simulink model "Simulink_EI"  (R2024b)
settings: Solver=ode23tb  StartTime=0.0  StopTime=20  FixedStep=0.00694  RelTol=1e-3
values from neighbouring files (symbols this model uses):
  beta = 1/1820.89    (= 0.000549181993421)    [Matlab_EI_1.m]
  Hco2 = 4003    [Matlab_EI_1.m]
  Ho2 = 94565    [Matlab_EI_1.m]
  phi = 0.2029    [Matlab_EI_1.m]
libraries: slpidlib x6
(part 1 of 2)
settings Model: Creator=julesmaugin  LastModifiedBy=julesmaugin

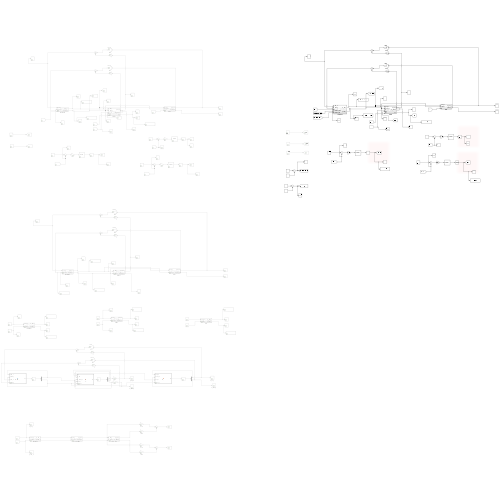
[thumbnail: Simulink's stored preview of the top-level diagram]
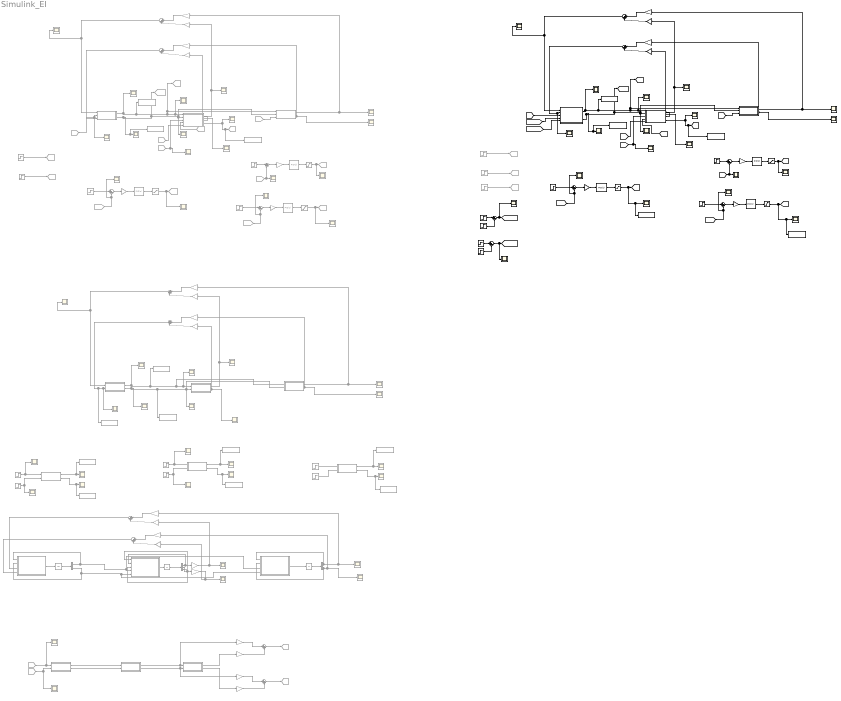
== system Simulink_EI ==
  1-phi{,1,4..7} (6 alike) : Gain  Commented=on  Gain=1-phi
  1-phi2 : Gain  Commented=on  Gain=0.7971
  1-phi3 : Gain  Commented=on  Gain=0.7971
  1-phi8 : Gain  Gain=1-phi
  1-phi9 : Gain  Gain=1-phi
  Algue : Subsystem  Commented=on
  Algue1 : Subsystem  Commented=on
  Algue2 : Subsystem  Commented=on
  Algue3 : Subsystem
  Blé : Subsystem  Commented=on
  Blé1 : Subsystem  Commented=on
  Blé2 : Subsystem  Commented=on
  Blé3 : Subsystem
  "C-IV a : algue" : Subsystem  Commented=on
  "C-IV b : blé" : Subsystem  Commented=on
  Demux : Demux  Commented=on  Outputs=2
  Demux1 : Demux  Commented=on  Outputs=3
  Demux2 : Demux  Commented=on  Outputs=2
  From : From  Commented=on  GotoTag=PO2e
  From1 : From  Commented=on  GotoTag=PCO2e
  From2 : From  Commented=on  GotoTag=Cx
  From3 : From  Commented=on  GotoTag=Lr
  From4 : From  Commented=on  GotoTag=P_CO2_c
  From5 : From  Commented=on  GotoTag=phi0
  From6 : From  Commented=on  GotoTag=Gc
  From7 : From  Commented=on  GotoTag=Gc
  From8 : From  Commented=on  GotoTag=Gc
  From9 : From  Commented=on  GotoTag=P_O2_c
  Gain : Gain  Commented=on  Gain=-10
  Gain1 : Gain  Commented=on  Gain=-5
  Gain2 : Gain  Commented=on
  Gain3 : Gain  Gain=-10
  Gain4 : Gain  Gain=-200
  Gain5 : Gain  Gain=10
  Goto : Goto  Commented=on  GotoTag=PO2e
  Goto1 : Goto  Commented=on  GotoTag=PCO2e
  Goto14 : Goto  Commented=on  GotoTag=phi0
  Goto17 : Goto  Commented=on  GotoTag=Gc
  Goto18 : Goto  Commented=on  GotoTag=Lr
  Goto2 : Goto  Commented=on  GotoTag=Lr
  Goto3 : Goto  Commented=on  GotoTag=Cx
  Goto4 : Goto  Commented=on  GotoTag=phi0
  Goto5 : Goto  Commented=on  GotoTag=P_CO2_c
  Goto6 : Goto  Commented=on  GotoTag=phi0
  Goto7 : Goto  Commented=on  GotoTag=Gc
  Goto8 : Goto  Commented=on  GotoTag=P_O2_c
  Goto9 : Goto  Commented=on  GotoTag=Gc
  Habitacle : Subsystem  Commented=on
  Habitacle1 : Subsystem  Commented=on
  Habitacle2 : Subsystem  Commented=on
  Habitacle3 : Subsystem  Commented=on
  Habitacle4 : Subsystem
  Integrator Limited : Integrator  Commented=on  InitialCondition=[20000;40]  LimitOutput=on  LowerSaturationLimit=0
  Integrator Limited1 : Integrator  Commented=on  InitialCondition=[0.212;18.79;1]  LimitOutput=on  LowerSaturationLimit=0
  Integrator Limited2 : Integrator  Commented=on  InitialCondition=[20000;20]  LimitOutput=on  LowerSaturationLimit=0
  MATLAB Function : MATLAB Function  Commented=on  TreatAsAtomicUnit=on
  MATLAB Function1 : MATLAB Function  Commented=on  TreatAsAtomicUnit=on
  MATLAB Function2 : MATLAB Function  Commented=on  TreatAsAtomicUnit=on
  Multiply : Gain  Commented=on  Gain=Ho2
  Multiply1 : Gain  Commented=on  Gain=Hco2
  PID Controller : slpidlib/PID Controller  Commented=on  Controller=PID  Form=Parallel  TimeDomain=Continuous-time  UseExternalTs=off  SampleTime=-1  IntegratorMethod=Forward Euler  FilterMethod=Forward Euler  ControllerParametersSource=internal  P=1  I=1  UseKiTs=off  D=0  UseExternalDerivativeSource=off  N=100  UseFilter=on  TunerSelectOption=Transfer Function Based (PID Tuner App)  InitialConditionSource=internal  InitialConditionForIntegrator=0  InitialConditionForFilter=0  DifferentiatorICPrevScaledInput=0  ExternalReset=none  TrackingMode=off  Kt=1  LimitOutput=off  SatLimitsSource=internal  UpperSaturationLimit=inf  LowerSaturationLimit=-inf  LinearizeAsGain=on  AntiWindupMode=none  Kb=1  LimitIntegrator=off  UpperIntegratorSaturationLimit=inf  LowerIntegratorSaturationLimit=-inf  POutMin=[]  POutMax=[]  IOutMin=[]  IOutMax=[]  DOutMin=[]  DOutMax=[]  NOutMin=[]  NOutMax=[]  SumOutMin=[]  SumOutMax=[]  SaturationOutMin=[]  SaturationOutMax=[]  PParamMin=[]  PParamMax=[]  IParamMin=[]  IParamMax=[]  DParamMin=[]  DParamMax=[]  NParamMin=[]  NParamMax=[]  KbParamMin=[]  KbParamMax=[]  KtParamMin=[]  KtParamMax=[]  KbOutMin=[]  KbOutMax=[]  KtOutMin=[]  KtOutMax=[]  IntegratorOutMin=[]  IntegratorOutMax=[]  FilterOutMin=[]  FilterOutMax=[]  SumI1OutMin=[]  SumI1OutMax=[]  SumI2OutMin=[]  SumI2OutMax=[]  SumI3OutMin=[]  SumI3OutMax=[]  SumI4OutMin=[]  SumI4OutMax=[]  SumDOutMin=[]  SumDOutMax=[]  DifferentiatorOutMin=[]  DifferentiatorOutMax=[]  FilterDiffOutCoefMin=[]  FilterDiffOutCoefMax=[]  ReciprocalOutMin=[]  ReciprocalOutMax=[]  SumDenOutMin=[]  SumDenOutMax=[]  SumNumOutMin=[]  SumNumOutMax=[]  DivideOutMin=[]  DivideOutMax=[]  UdiffTsProdOutMin=[]  UdiffTsProdOutMax=[]  NTsProdOutMin=[]  NTsProdOutMax=[]  UintegralTsProdOutMin=[]  UintegralTsProdOutMax=[]  UngainTsProdOutMin=[]  UngainTsProdOutMax=[]  ClampingZeroOutDataTypeStr=Inherit: Inherit via back propagation  ClampingZeroOutMin=[]  ClampingZeroOutMax=[]  FilterDenConstantOutDataTypeStr=Inherit: Inherit via back propagation  FilterDenConstantOutMin=[]  FilterDenConstantOutMax=[]  PCopyOutDataTypeStr=Inherit: Inherit via back propagation  PCopyOutMin=[]  PCopyOutMax=[]  NCopyOutDataTypeStr=Inherit: Inherit via back propagation  NCopyOutMin=[]  NCopyOutMax=[]  IntegratorContinuousStateAttributes=''  IntegratorStateMustResolveToSignalObject=off  IntegratorRTWStateStorageClass=Auto  FilterContinuousStateAttributes=''  FilterStateMustResolveToSignalObject=off  FilterRTWStateStorageClass=Auto  ParallelPVariant=InternalParameters  IdealPVariant=Disabled  IVariant=InternalParameters  DVariant=InternalParameters  IntegratorVariant=Continuous  SatVariant=Disabled  AWVariant=Passthrough  PCopyVariant=Disabled  TRVariant=Disabled  FdbkBlocksVariant=Forward  IdealPFdbkVariant=Disabled  SatFdbkVariant=Disabled  DerivativeFilterVariant=ContFilter  NVariant=InternalParameters  NCopyVariant=Disabled  FilterICVariant=InternalICsFilter  IntegratorICVariant=InternalICs  ExternalResetVariant=Disabled  TRSumVariant=Passthrough  SumFdbkVariant=Disabled  SumVariant=Sum_PID  TsampFilterVariant=InternalTs  TsampNgainVariant=Passthrough  TsampIntegralVariant=Disabled_SignalSpec  ExternalSaturationOutDataTypeStr=Inherit: Same as second input  DerivativeSourceVariant=ErrorSignal  PreIntVariant=InternalPreInt
  PID Controller1 : slpidlib/PID Controller  Commented=on  Controller=PID  Form=Parallel  TimeDomain=Continuous-time  UseExternalTs=off  SampleTime=-1  IntegratorMethod=Forward Euler  FilterMethod=Forward Euler  ControllerParametersSource=internal  P=1  I=10  UseKiTs=off  D=0  UseExternalDerivativeSource=off  N=100  UseFilter=on  TunerSelectOption=Transfer Function Based (PID Tuner App)  InitialConditionSource=internal  InitialConditionForIntegrator=0  InitialConditionForFilter=0  DifferentiatorICPrevScaledInput=0  ExternalReset=none  TrackingMode=off  Kt=1  LimitOutput=off  SatLimitsSource=internal  UpperSaturationLimit=inf  LowerSaturationLimit=-inf  LinearizeAsGain=on  AntiWindupMode=none  Kb=1  LimitIntegrator=off  UpperIntegratorSaturationLimit=inf  LowerIntegratorSaturationLimit=-inf  POutMin=[]  POutMax=[]  IOutMin=[]  IOutMax=[]  DOutMin=[]  DOutMax=[]  NOutMin=[]  NOutMax=[]  SumOutMin=[]  SumOutMax=[]  SaturationOutMin=[]  SaturationOutMax=[]  PParamMin=[]  PParamMax=[]  IParamMin=[]  IParamMax=[]  DParamMin=[]  DParamMax=[]  NParamMin=[]  NParamMax=[]  KbParamMin=[]  KbParamMax=[]  KtParamMin=[]  KtParamMax=[]  KbOutMin=[]  KbOutMax=[]  KtOutMin=[]  KtOutMax=[]  IntegratorOutMin=[]  IntegratorOutMax=[]  FilterOutMin=[]  FilterOutMax=[]  SumI1OutMin=[]  SumI1OutMax=[]  SumI2OutMin=[]  SumI2OutMax=[]  SumI3OutMin=[]  SumI3OutMax=[]  SumI4OutMin=[]  SumI4OutMax=[]  SumDOutMin=[]  SumDOutMax=[]  DifferentiatorOutMin=[]  DifferentiatorOutMax=[]  FilterDiffOutCoefMin=[]  FilterDiffOutCoefMax=[]  ReciprocalOutMin=[]  ReciprocalOutMax=[]  SumDenOutMin=[]  SumDenOutMax=[]  SumNumOutMin=[]  SumNumOutMax=[]  DivideOutMin=[]  DivideOutMax=[]  UdiffTsProdOutMin=[]  UdiffTsProdOutMax=[]  NTsProdOutMin=[]  NTsProdOutMax=[]  UintegralTsProdOutMin=[]  UintegralTsProdOutMax=[]  UngainTsProdOutMin=[]  UngainTsProdOutMax=[]  ClampingZeroOutDataTypeStr=Inherit: Inherit via back propagation  ClampingZeroOutMin=[]  ClampingZeroOutMax=[]  FilterDenConstantOutDataTypeStr=Inherit: Inherit via back propagation  FilterDenConstantOutMin=[]  FilterDenConstantOutMax=[]  PCopyOutDataTypeStr=Inherit: Inherit via back propagation  PCopyOutMin=[]  PCopyOutMax=[]  NCopyOutDataTypeStr=Inherit: Inherit via back propagation  NCopyOutMin=[]  NCopyOutMax=[]  IntegratorContinuousStateAttributes=''  IntegratorStateMustResolveToSignalObject=off  IntegratorRTWStateStorageClass=Auto  FilterContinuousStateAttributes=''  FilterStateMustResolveToSignalObject=off  FilterRTWStateStorageClass=Auto  ParallelPVariant=InternalParameters  IdealPVariant=Disabled  IVariant=InternalParameters  DVariant=InternalParameters  IntegratorVariant=Continuous  SatVariant=Disabled  AWVariant=Passthrough  PCopyVariant=Disabled  TRVariant=Disabled  FdbkBlocksVariant=Forward  IdealPFdbkVariant=Disabled  SatFdbkVariant=Disabled  DerivativeFilterVariant=ContFilter  NVariant=InternalParameters  NCopyVariant=Disabled  FilterICVariant=InternalICsFilter  IntegratorICVariant=InternalICs  ExternalResetVariant=Disabled  TRSumVariant=Passthrough  SumFdbkVariant=Disabled  SumVariant=Sum_PID  TsampFilterVariant=InternalTs  TsampNgainVariant=Passthrough  TsampIntegralVariant=Disabled_SignalSpec  ExternalSaturationOutDataTypeStr=Inherit: Same as second input  DerivativeSourceVariant=ErrorSignal  PreIntVariant=InternalPreInt
  PID Controller2 : slpidlib/PID Controller  Commented=on  Controller=PID  Form=Parallel  TimeDomain=Continuous-time  UseExternalTs=off  SampleTime=-1  IntegratorMethod=Forward Euler  FilterMethod=Forward Euler  ControllerParametersSource=internal  P=1  I=0  UseKiTs=off  D=0  UseExternalDerivativeSource=off  N=100  UseFilter=on  TunerSelectOption=Transfer Function Based (PID Tuner App)  InitialConditionSource=internal  InitialConditionForIntegrator=0  InitialConditionForFilter=0  DifferentiatorICPrevScaledInput=0  ExternalReset=none  TrackingMode=off  Kt=1  LimitOutput=off  SatLimitsSource=internal  UpperSaturationLimit=inf  LowerSaturationLimit=-inf  LinearizeAsGain=on  AntiWindupMode=none  Kb=1  LimitIntegrator=off  UpperIntegratorSaturationLimit=inf  LowerIntegratorSaturationLimit=-inf  POutMin=[]  POutMax=[]  IOutMin=[]  IOutMax=[]  DOutMin=[]  DOutMax=[]  NOutMin=[]  NOutMax=[]  SumOutMin=[]  SumOutMax=[]  SaturationOutMin=[]  SaturationOutMax=[]  PParamMin=[]  PParamMax=[]  IParamMin=[]  IParamMax=[]  DParamMin=[]  DParamMax=[]  NParamMin=[]  NParamMax=[]  KbParamMin=[]  KbParamMax=[]  KtParamMin=[]  KtParamMax=[]  KbOutMin=[]  KbOutMax=[]  KtOutMin=[]  KtOutMax=[]  IntegratorOutMin=[]  IntegratorOutMax=[]  FilterOutMin=[]  FilterOutMax=[]  SumI1OutMin=[]  SumI1OutMax=[]  SumI2OutMin=[]  SumI2OutMax=[]  SumI3OutMin=[]  SumI3OutMax=[]  SumI4OutMin=[]  SumI4OutMax=[]  SumDOutMin=[]  SumDOutMax=[]  DifferentiatorOutMin=[]  DifferentiatorOutMax=[]  FilterDiffOutCoefMin=[]  FilterDiffOutCoefMax=[]  ReciprocalOutMin=[]  ReciprocalOutMax=[]  SumDenOutMin=[]  SumDenOutMax=[]  SumNumOutMin=[]  SumNumOutMax=[]  DivideOutMin=[]  DivideOutMax=[]  UdiffTsProdOutMin=[]  UdiffTsProdOutMax=[]  NTsProdOutMin=[]  NTsProdOutMax=[]  UintegralTsProdOutMin=[]  UintegralTsProdOutMax=[]  UngainTsProdOutMin=[]  UngainTsProdOutMax=[]  ClampingZeroOutDataTypeStr=Inherit: Inherit via back propagation  ClampingZeroOutMin=[]  ClampingZeroOutMax=[]  FilterDenConstantOutDataTypeStr=Inherit: Inherit via back propagation  FilterDenConstantOutMin=[]  FilterDenConstantOutMax=[]  PCopyOutDataTypeStr=Inherit: Inherit via back propagation  PCopyOutMin=[]  PCopyOutMax=[]  NCopyOutDataTypeStr=Inherit: Inherit via back propagation  NCopyOutMin=[]  NCopyOutMax=[]  IntegratorContinuousStateAttributes=''  IntegratorStateMustResolveToSignalObject=off  IntegratorRTWStateStorageClass=Auto  FilterContinuousStateAttributes=''  FilterStateMustResolveToSignalObject=off  FilterRTWStateStorageClass=Auto  ParallelPVariant=InternalParameters  IdealPVariant=Disabled  IVariant=InternalParameters  DVariant=InternalParameters  IntegratorVariant=Continuous  SatVariant=Disabled  AWVariant=Passthrough  PCopyVariant=Disabled  TRVariant=Disabled  FdbkBlocksVariant=Forward  IdealPFdbkVariant=Disabled  SatFdbkVariant=Disabled  DerivativeFilterVariant=ContFilter  NVariant=InternalParameters  NCopyVariant=Disabled  FilterICVariant=InternalICsFilter  IntegratorICVariant=InternalICs  ExternalResetVariant=Disabled  TRSumVariant=Passthrough  SumFdbkVariant=Disabled  SumVariant=Sum_PID  TsampFilterVariant=InternalTs  TsampNgainVariant=Passthrough  TsampIntegralVariant=Disabled_SignalSpec  ExternalSaturationOutDataTypeStr=Inherit: Same as second input  DerivativeSourceVariant=ErrorSignal  PreIntVariant=InternalPreInt
  PID Controller3 : slpidlib/PID Controller  Controller=PID  Form=Parallel  TimeDomain=Continuous-time  UseExternalTs=off  SampleTime=-1  IntegratorMethod=Forward Euler  FilterMethod=Forward Euler  ControllerParametersSource=internal  P=1  I=1  UseKiTs=off  D=0  UseExternalDerivativeSource=off  N=100  UseFilter=on  TunerSelectOption=Transfer Function Based (PID Tuner App)  InitialConditionSource=internal  InitialConditionForIntegrator=0  InitialConditionForFilter=0  DifferentiatorICPrevScaledInput=0  ExternalReset=none  TrackingMode=off  Kt=1  LimitOutput=off  SatLimitsSource=internal  UpperSaturationLimit=inf  LowerSaturationLimit=-inf  LinearizeAsGain=on  AntiWindupMode=none  Kb=1  LimitIntegrator=off  UpperIntegratorSaturationLimit=inf  LowerIntegratorSaturationLimit=-inf  POutMin=[]  POutMax=[]  IOutMin=[]  IOutMax=[]  DOutMin=[]  DOutMax=[]  NOutMin=[]  NOutMax=[]  SumOutMin=[]  SumOutMax=[]  SaturationOutMin=[]  SaturationOutMax=[]  PParamMin=[]  PParamMax=[]  IParamMin=[]  IParamMax=[]  DParamMin=[]  DParamMax=[]  NParamMin=[]  NParamMax=[]  KbParamMin=[]  KbParamMax=[]  KtParamMin=[]  KtParamMax=[]  KbOutMin=[]  KbOutMax=[]  KtOutMin=[]  KtOutMax=[]  IntegratorOutMin=[]  IntegratorOutMax=[]  FilterOutMin=[]  FilterOutMax=[]  SumI1OutMin=[]  SumI1OutMax=[]  SumI2OutMin=[]  SumI2OutMax=[]  SumI3OutMin=[]  SumI3OutMax=[]  SumI4OutMin=[]  SumI4OutMax=[]  SumDOutMin=[]  SumDOutMax=[]  DifferentiatorOutMin=[]  DifferentiatorOutMax=[]  FilterDiffOutCoefMin=[]  FilterDiffOutCoefMax=[]  ReciprocalOutMin=[]  ReciprocalOutMax=[]  SumDenOutMin=[]  SumDenOutMax=[]  SumNumOutMin=[]  SumNumOutMax=[]  DivideOutMin=[]  DivideOutMax=[]  UdiffTsProdOutMin=[]  UdiffTsProdOutMax=[]  NTsProdOutMin=[]  NTsProdOutMax=[]  UintegralTsProdOutMin=[]  UintegralTsProdOutMax=[]  UngainTsProdOutMin=[]  UngainTsProdOutMax=[]  ClampingZeroOutDataTypeStr=Inherit: Inherit via back propagation  ClampingZeroOutMin=[]  ClampingZeroOutMax=[]  FilterDenConstantOutDataTypeStr=Inherit: Inherit via back propagation  FilterDenConstantOutMin=[]  FilterDenConstantOutMax=[]  PCopyOutDataTypeStr=Inherit: Inherit via back propagation  PCopyOutMin=[]  PCopyOutMax=[]  NCopyOutDataTypeStr=Inherit: Inherit via back propagation  NCopyOutMin=[]  NCopyOutMax=[]  IntegratorContinuousStateAttributes=''  IntegratorStateMustResolveToSignalObject=off  IntegratorRTWStateStorageClass=Auto  FilterContinuousStateAttributes=''  FilterStateMustResolveToSignalObject=off  FilterRTWStateStorageClass=Auto  ParallelPVariant=InternalParameters  IdealPVariant=Disabled  IVariant=InternalParameters  DVariant=InternalParameters  IntegratorVariant=Continuous  SatVariant=Disabled  AWVariant=Passthrough  PCopyVariant=Disabled  TRVariant=Disabled  FdbkBlocksVariant=Forward  IdealPFdbkVariant=Disabled  SatFdbkVariant=Disabled  DerivativeFilterVariant=ContFilter  NVariant=InternalParameters  NCopyVariant=Disabled  FilterICVariant=InternalICsFilter  IntegratorICVariant=InternalICs  ExternalResetVariant=Disabled  TRSumVariant=Passthrough  SumFdbkVariant=Disabled  SumVariant=Sum_PID  TsampFilterVariant=InternalTs  TsampNgainVariant=Passthrough  TsampIntegralVariant=Disabled_SignalSpec  ExternalSaturationOutDataTypeStr=Inherit: Same as second input  DerivativeSourceVariant=ErrorSignal  PreIntVariant=InternalPreInt
  PID Controller4 : slpidlib/PID Controller  Controller=PID  Form=Parallel  TimeDomain=Continuous-time  UseExternalTs=off  SampleTime=-1  IntegratorMethod=Forward Euler  FilterMethod=Forward Euler  ControllerParametersSource=internal  P=1  I=1  UseKiTs=off  D=0  UseExternalDerivativeSource=off  N=100  UseFilter=on  TunerSelectOption=Transfer Function Based (PID Tuner App)  InitialConditionSource=internal  InitialConditionForIntegrator=0  InitialConditionForFilter=0  DifferentiatorICPrevScaledInput=0  ExternalReset=none  TrackingMode=off  Kt=1  LimitOutput=off  SatLimitsSource=internal  UpperSaturationLimit=inf  LowerSaturationLimit=-inf  LinearizeAsGain=on  AntiWindupMode=none  Kb=1  LimitIntegrator=off  UpperIntegratorSaturationLimit=inf  LowerIntegratorSaturationLimit=-inf  POutMin=[]  POutMax=[]  IOutMin=[]  IOutMax=[]  DOutMin=[]  DOutMax=[]  NOutMin=[]  NOutMax=[]  SumOutMin=[]  SumOutMax=[]  SaturationOutMin=[]  SaturationOutMax=[]  PParamMin=[]  PParamMax=[]  IParamMin=[]  IParamMax=[]  DParamMin=[]  DParamMax=[]  NParamMin=[]  NParamMax=[]  KbParamMin=[]  KbParamMax=[]  KtParamMin=[]  KtParamMax=[]  KbOutMin=[]  KbOutMax=[]  KtOutMin=[]  KtOutMax=[]  IntegratorOutMin=[]  IntegratorOutMax=[]  FilterOutMin=[]  FilterOutMax=[]  SumI1OutMin=[]  SumI1OutMax=[]  SumI2OutMin=[]  SumI2OutMax=[]  SumI3OutMin=[]  SumI3OutMax=[]  SumI4OutMin=[]  SumI4OutMax=[]  SumDOutMin=[]  SumDOutMax=[]  DifferentiatorOutMin=[]  DifferentiatorOutMax=[]  FilterDiffOutCoefMin=[]  FilterDiffOutCoefMax=[]  ReciprocalOutMin=[]  ReciprocalOutMax=[]  SumDenOutMin=[]  SumDenOutMax=[]  SumNumOutMin=[]  SumNumOutMax=[]  DivideOutMin=[]  DivideOutMax=[]  UdiffTsProdOutMin=[]  UdiffTsProdOutMax=[]  NTsProdOutMin=[]  NTsProdOutMax=[]  UintegralTsProdOutMin=[]  UintegralTsProdOutMax=[]  UngainTsProdOutMin=[]  UngainTsProdOutMax=[]  ClampingZeroOutDataTypeStr=Inherit: Inherit via back propagation  ClampingZeroOutMin=[]  ClampingZeroOutMax=[]  FilterDenConstantOutDataTypeStr=Inherit: Inherit via back propagation  FilterDenConstantOutMin=[]  FilterDenConstantOutMax=[]  PCopyOutDataTypeStr=Inherit: Inherit via back propagation  PCopyOutMin=[]  PCopyOutMax=[]  NCopyOutDataTypeStr=Inherit: Inherit via back propagation  NCopyOutMin=[]  NCopyOutMax=[]  IntegratorContinuousStateAttributes=''  IntegratorStateMustResolveToSignalObject=off  IntegratorRTWStateStorageClass=Auto  FilterContinuousStateAttributes=''  FilterStateMustResolveToSignalObject=off  FilterRTWStateStorageClass=Auto  ParallelPVariant=InternalParameters  IdealPVariant=Disabled  IVariant=InternalParameters  DVariant=InternalParameters  IntegratorVariant=Continuous  SatVariant=Disabled  AWVariant=Passthrough  PCopyVariant=Disabled  TRVariant=Disabled  FdbkBlocksVariant=Forward  IdealPFdbkVariant=Disabled  SatFdbkVariant=Disabled  DerivativeFilterVariant=ContFilter  NVariant=InternalParameters  NCopyVariant=Disabled  FilterICVariant=InternalICsFilter  IntegratorICVariant=InternalICs  ExternalResetVariant=Disabled  TRSumVariant=Passthrough  SumFdbkVariant=Disabled  SumVariant=Sum_PID  TsampFilterVariant=InternalTs  TsampNgainVariant=Passthrough  TsampIntegralVariant=Disabled_SignalSpec  ExternalSaturationOutDataTypeStr=Inherit: Same as second input  DerivativeSourceVariant=ErrorSignal  PreIntVariant=InternalPreInt
  PID Controller5 : slpidlib/PID Controller  Controller=PID  Form=Parallel  TimeDomain=Continuous-time  UseExternalTs=off  SampleTime=-1  IntegratorMethod=Forward Euler  FilterMethod=Forward Euler  ControllerParametersSource=internal  P=1  I=1  UseKiTs=off  D=0  UseExternalDerivativeSource=off  N=100  UseFilter=on  TunerSelectOption=Transfer Function Based (PID Tuner App)  InitialConditionSource=internal  InitialConditionForIntegrator=0  InitialConditionForFilter=0  DifferentiatorICPrevScaledInput=0  ExternalReset=none  TrackingMode=off  Kt=1  LimitOutput=off  SatLimitsSource=internal  UpperSaturationLimit=inf  LowerSaturationLimit=-inf  LinearizeAsGain=on  AntiWindupMode=none  Kb=1  LimitIntegrator=off  UpperIntegratorSaturationLimit=inf  LowerIntegratorSaturationLimit=-inf  POutMin=[]  POutMax=[]  IOutMin=[]  IOutMax=[]  DOutMin=[]  DOutMax=[]  NOutMin=[]  NOutMax=[]  SumOutMin=[]  SumOutMax=[]  SaturationOutMin=[]  SaturationOutMax=[]  PParamMin=[]  PParamMax=[]  IParamMin=[]  IParamMax=[]  DParamMin=[]  DParamMax=[]  NParamMin=[]  NParamMax=[]  KbParamMin=[]  KbParamMax=[]  KtParamMin=[]  KtParamMax=[]  KbOutMin=[]  KbOutMax=[]  KtOutMin=[]  KtOutMax=[]  IntegratorOutMin=[]  IntegratorOutMax=[]  FilterOutMin=[]  FilterOutMax=[]  SumI1OutMin=[]  SumI1OutMax=[]  SumI2OutMin=[]  SumI2OutMax=[]  SumI3OutMin=[]  SumI3OutMax=[]  SumI4OutMin=[]  SumI4OutMax=[]  SumDOutMin=[]  SumDOutMax=[]  DifferentiatorOutMin=[]  DifferentiatorOutMax=[]  FilterDiffOutCoefMin=[]  FilterDiffOutCoefMax=[]  ReciprocalOutMin=[]  ReciprocalOutMax=[]  SumDenOutMin=[]  SumDenOutMax=[]  SumNumOutMin=[]  SumNumOutMax=[]  DivideOutMin=[]  DivideOutMax=[]  UdiffTsProdOutMin=[]  UdiffTsProdOutMax=[]  NTsProdOutMin=[]  NTsProdOutMax=[]  UintegralTsProdOutMin=[]  UintegralTsProdOutMax=[]  UngainTsProdOutMin=[]  UngainTsProdOutMax=[]  ClampingZeroOutDataTypeStr=Inherit: Inherit via back propagation  ClampingZeroOutMin=[]  ClampingZeroOutMax=[]  FilterDenConstantOutDataTypeStr=Inherit: Inherit via back propagation  FilterDenConstantOutMin=[]  FilterDenConstantOutMax=[]  PCopyOutDataTypeStr=Inherit: Inherit via back propagation  PCopyOutMin=[]  PCopyOutMax=[]  NCopyOutDataTypeStr=Inherit: Inherit via back propagation  NCopyOutMin=[]  NCopyOutMax=[]  IntegratorContinuousStateAttributes=''  IntegratorStateMustResolveToSignalObject=off  IntegratorRTWStateStorageClass=Auto  FilterContinuousStateAttributes=''  FilterStateMustResolveToSignalObject=off  FilterRTWStateStorageClass=Auto  ParallelPVariant=InternalParameters  IdealPVariant=Disabled  IVariant=InternalParameters  DVariant=InternalParameters  IntegratorVariant=Continuous  SatVariant=Disabled  AWVariant=Passthrough  PCopyVariant=Disabled  TRVariant=Disabled  FdbkBlocksVariant=Forward  IdealPFdbkVariant=Disabled  SatFdbkVariant=Disabled  DerivativeFilterVariant=ContFilter  NVariant=InternalParameters  NCopyVariant=Disabled  FilterICVariant=InternalICsFilter  IntegratorICVariant=InternalICs  ExternalResetVariant=Disabled  TRSumVariant=Passthrough  SumFdbkVariant=Disabled  SumVariant=Sum_PID  TsampFilterVariant=InternalTs  TsampNgainVariant=Passthrough  TsampIntegralVariant=Disabled_SignalSpec  ExternalSaturationOutDataTypeStr=Inherit: Same as second input  DerivativeSourceVariant=ErrorSignal  PreIntVariant=InternalPreInt
  P_02_a : Scope  Commented=on
  P_02_b : Scope  Commented=on
  P_02_e : Scope  Commented=on
  P_C02_a : Scope  Commented=on
  P_C02_b : Scope  Commented=on
  P_C02_e : Scope  Commented=on
  Saturation : Saturate  Commented=on  UpperLimit=inf  LowerLimit=0
  Saturation1 : Saturate  Commented=on  UpperLimit=500  LowerLimit=10
  Saturation2 : Saturate  Commented=on  UpperLimit=50000  LowerLimit=7000
  Saturation3 : Saturate  UpperLimit=inf  LowerLimit=0
  Saturation4 : Saturate  UpperLimit=inf  LowerLimit=7000
  Saturation5 : Saturate  UpperLimit=350  LowerLimit=10
  Scope{,1..37} (38 alike) : Scope  Commented=on
  Scope{38..57} (20 alike) : Scope
  Step : Step  Commented=on  Before=21000  After=21000  SampleTime=0
  Step1 : Step  Commented=on  Before=18  After=18  SampleTime=0
  Step10 : Step  Commented=on  Before=13680  After=13680  SampleTime=0
  Step11 : Step  Commented=on  Before=13680  After=13680  SampleTime=0
  Step12 : Step  Before=1  SampleTime=0
  Step13 : Step  Before=40  After=40  SampleTime=0
  Step14 : Step  Commented=on  Before=350  After=350  SampleTime=0
  Step15 : Step  Before=20000  After=20000  SampleTime=0
  Step16 : Step  Commented=on  Before=0.52992  After=0.52992  SampleTime=0
  Step17 : Step  Time=10  Before=0.982*24  After=56.6  SampleTime=0
  Step18 : Step  Time=10  Before=-1.065*24  After=-55.9  SampleTime=0
  Step19 : Step  Time=10+30/(60*24)  After=56.6-0.982*24  SampleTime=0
  Step2 : Step  Commented=on  Before=20000  After=20000  SampleTime=0
  Step20 : Step  Time=10+30/(60*24)  After=-55.9+1.065*24  SampleTime=0
  Step3 : Step  Commented=on  Before=40  After=40  SampleTime=0
  Step4 : Step  Commented=on  Before=20000  After=20000  SampleTime=0
  Step5 : Step  Commented=on  Before=40  After=40  SampleTime=0
  Step6 : Step  Commented=on  Before=1  SampleTime=0
  Step7 : Step  Commented=on  Before=40  After=40  SampleTime=0
  Step8 : Step  Commented=on  Before=350  After=350  SampleTime=0
  Step9 : Step  Commented=on  Before=20000  After=20000  SampleTime=0
  Sum{,1..7} (8 alike) : Sum  Commented=on  Inputs=|++
  Sum10 : Sum  Commented=on  Inputs=|+-
  Sum{11,14..17} (5 alike) : Sum  Inputs=|+-
  Sum12 : Sum  Inputs=|++
  Sum13 : Sum  Inputs=|++
  Sum8 : Sum  Commented=on  Inputs=|+-
  Sum9 : Sum  Commented=on  Inputs=|+-
  To Workspace : ToWorkspace  Commented=on  VariableName=P_O2_c  SaveFormat=Timeseries  SampleTime=-1
  To Workspace1 : ToWorkspace  Commented=on  VariableName=P_CO2_c  SaveFormat=Timeseries  SampleTime=-1
  To Workspace10 : ToWorkspace  Commented=on  VariableName=P_CO2_c  SaveFormat=Timeseries  SampleTime=-1
  To Workspace11 : ToWorkspace  Commented=on  VariableName=P_O2_c  SaveFormat=Timeseries  SampleTime=-1
  To Workspace12 : ToWorkspace  VariableName=P_CO2_c  SaveFormat=Timeseries  SampleTime=-1
  To Workspace13 : ToWorkspace  VariableName=P_O2_c  SaveFormat=Timeseries  SampleTime=-1
  To Workspace14 : ToWorkspace  VariableName=Cx  SaveFormat=Timeseries  SampleTime=-1
  To Workspace15 : ToWorkspace  VariableName=phi0  SaveFormat=Timeseries  SampleTime=-1
  To Workspace16 : ToWorkspace  VariableName=Gc  SaveFormat=Timeseries  SampleTime=-1
  To Workspace2 : ToWorkspace  Commented=on  VariableName=P_O2_a  SaveFormat=Timeseries  SampleTime=-1
  To Workspace3 : ToWorkspace  Commented=on  VariableName=P_CO2_a  SaveFormat=Timeseries  SampleTime=-1
  To Workspace4 : ToWorkspace  Commented=on  VariableName=P_02_b  SaveFormat=Timeseries  SampleTime=-1
  To Workspace5 : ToWorkspace  Commented=on  VariableName=P_CO2_b  SaveFormat=Timeseries  SampleTime=-1
  To Workspace6 : ToWorkspace  Commented=on  VariableName=P_O2_c  SaveFormat=Timeseries  SampleTime=-1
  To Workspace7 : ToWorkspace  Commented=on  VariableName=P_CO2_c  SaveFormat=Timeseries  SampleTime=-1
  To Workspace8 : ToWorkspace  Commented=on  VariableName=P_CO2_e  SaveFormat=Timeseries  SampleTime=-1
  To Workspace9 : ToWorkspace  Commented=on  VariableName=Cx  SaveFormat=Timeseries  SampleTime=-1
  phi{,1,4..7} (6 alike) : Gain  Commented=on  Gain=phi
  phi2 : Gain  Commented=on  Gain=0.2029
  phi3 : Gain  Commented=on  Gain=0.2029
  phi8 : Gain  Gain=phi
  phi9 : Gain  Gain=phi
  wires:
  MATLAB Function/1(dx) -> Integrator Limited/1
  Sum1/1 -> MATLAB Function/4(P_CO2_e)
  Integrator Limited/1 -> Demux/1
  Demux/1 -> MATLAB Function1/4(P_O2_c), MATLAB Function2/3(P_O2_c), MATLAB Function/1(P_O2_c)
  Demux/2 -> MATLAB Function/2(P_CO2_c), MATLAB Function2/4(P_CO2_c), MATLAB Function1/5(P_CO2_c)
  MATLAB Function1/1(dx) -> Integrator Limited1/1
  Integrator Limited1/1 -> Demux1/1
  Demux1/1 -> MATLAB Function1/2(C_O2), Multiply/1
  Demux1/2 -> MATLAB Function1/3(C_CO2_CT), Multiply1/1
  MATLAB Function2/1(dx) -> Integrator Limited2/1
  Integrator Limited2/1 -> Demux2/1
  Demux2/1 -> MATLAB Function2/1(P_O2_b), 1-phi/1, P_02_b/1
  Demux2/2 -> 1-phi1/1, P_C02_b/1, MATLAB Function2/2(P_CO2_b)
  phi/1 -> Sum/2
  1-phi/1 -> Sum/1
  Sum/1 -> MATLAB Function/3(P_O2_e)
  1-phi1/1 -> Sum1/1
  phi1/1 -> Sum1/2
  Habitacle/1(P_O2_c) -> "C-IV a : algue"/1(P_O2_c)
  Habitacle/2(P_CO2_c) -> "C-IV a : algue"/2(P_CO2_c)
  "C-IV a : algue"/1(P_O2_a) -> phi2/1, "C-IV b : blé"/1(P_O2_c)
  "C-IV a : algue"/2(P_CO2_a) -> phi3/1, "C-IV b : blé"/2(P_CO2_c)
  phi2/1 -> Sum2/1
  1-phi2/1 -> Sum2/2
  "C-IV b : blé"/1(P_O2_b) -> 1-phi2/1
  1-phi3/1 -> Sum3/2
  phi3/1 -> Sum3/1
  "C-IV b : blé"/2(P_CO2_b) -> 1-phi3/1
  Sum2/1 -> Goto/1
  From/1 -> P_02_e/1, Habitacle/1(P_O2_e)
  From1/1 -> P_C02_e/1, Habitacle/2(P_CO2_e)
  Sum3/1 -> Goto1/1
  Demux1/3 -> MATLAB Function1/1(Cx)
  Multiply/1 -> phi/1, P_02_a/1
  Multiply1/1 -> phi1/1, P_C02_a/1
  Step/1 -> Scope3/1, Habitacle1/1(P_O2_e)
  Step1/1 -> Scope2/1, Habitacle1/2(P_CO2_e)
  Habitacle1/1(P_O2_c) -> To Workspace/1, Scope/1
  Habitacle1/2(P_CO2_c) -> To Workspace1/1, Scope1/1
  Step2/1 -> Scope6/1, Algue/1(P_O2_c)
  Step3/1 -> Scope7/1, Algue/2(P_CO2_c)
  Algue/1(P_O2_a) -> To Workspace2/1, Scope4/1
  Algue/2(P_CO2_a) -> To Workspace3/1, Scope5/1
  Step4/1 -> Blé/1(P_O2_c)
  Step5/1 -> Blé/2(P_CO2_c)
  Blé/2(P_CO2_b) -> To Workspace5/1, Scope9/1
  Blé/1(P_O2_b) -> To Workspace4/1, Scope8/1
  Habitacle2/2(P_CO2_c) -> To Workspace7/1, Scope17/1, Algue1/2(P_CO2_c), Blé1/2(P_CO2_c), Scope11/1
  Blé1/2(P_CO2_b) -> 1-phi5/1, Scope19/1
  Habitacle2/1(P_O2_c) -> To Workspace6/1, Blé1/1(P_O2_c), Scope16/1, Algue1/1(P_O2_c), Scope10/1
  Algue1/1(P_O2_a) -> phi4/1, Scope14/1
  Algue1/2(P_CO2_a) -> phi5/1, Scope15/1
  Blé1/1(P_O2_b) -> 1-phi4/1, Scope18/1
  1-phi4/1 -> Sum4/1
  phi4/1 -> Sum4/2
  phi5/1 -> Sum5/2
  1-phi5/1 -> Sum5/1
  Sum5/1 -> To Workspace8/1, Scope12/1, Habitacle2/2(P_CO2_e)
  Sum4/1 -> Scope13/1, Habitacle2/1(P_O2_e)
  1-phi6/1 -> Sum6/1
  Algue2/2(P_CO2_a) -> Scope25/1, phi7/1
  Algue2/1(P_O2_a) -> phi6/1, Scope24/1
  Sum7/1 -> Scope22/1, Habitacle3/2(P_CO2_e)
  Blé2/1(P_O2_b) -> 1-phi6/1, Scope28/1
  Habitacle3/2(P_CO2_c) -> Goto5/1, Scope27/1, Algue2/2(P_CO2_c), Blé2/2(P_CO2_c), To Workspace10/1, Scope21/1
  Habitacle3/1(P_O2_c) -> To Workspace11/1, Blé2/1(P_O2_c), Goto8/1, Scope26/1, Algue2/1(P_O2_c), Scope20/1
  Blé2/2(P_CO2_b) -> 1-phi7/1, Scope29/1
  Sum6/1 -> Scope23/1, Habitacle3/1(P_O2_e)
  phi6/1 -> Sum6/2
  phi7/1 -> Sum7/2
  1-phi7/1 -> Sum7/1
  Step6/1 -> Sum8/1
  From2/1 -> Sum8/2, Scope32/1
  Sum8/1 -> Gain/1
  Gain/1 -> PID Controller/1
  PID Controller/1 -> Saturation/1
  Saturation/1 -> Scope31/1, Goto2/1
  From3/1 -> Scope30/1, Algue2/3(Lr)
  Algue2/3(Cx) -> Scope33/1, To Workspace9/1, Goto3/1
  Saturation1/1 -> Scope34/1, Goto4/1
  From4/1 -> Sum9/2, Scope35/1
  Gain1/1 -> PID Controller1/1
  PID Controller1/1 -> Saturation1/1
  Sum9/1 -> Gain1/1
  Step7/1 -> Sum9/1
  From5/1 -> Algue2/4(phi0)
  Step8/1 -> Goto6/1
  From6/1 -> Habitacle3/3(Gc)
  From7/1 -> Algue2/5(Gc)
  From8/1 -> Blé2/3(Gc)
  Gain2/1 -> PID Controller2/1
  From9/1 -> Sum10/2, Scope37/1
  Step9/1 -> Sum10/1
  Sum10/1 -> Gain2/1
  PID Controller2/1 -> Saturation2/1
  Saturation2/1 -> Scope36/1, Goto7/1
  Step10/1 -> Goto9/1
  1-phi8/1 -> Sum12/1
  PID Controller3/1 -> Saturation3/1
  Gain4/1 -> PID Controller4/1
  [Lr] -> Scope48/1, Algue3/3(Lr)
  Sum14/1 -> Gain3/1
  Step12/1 -> Sum14/1
  Step15/1 -> Sum11/1
  1-phi9/1 -> Sum13/1
  Step13/1 -> Sum15/1
  Algue3/3(Cx) -> Scope51/1, To Workspace14/1, [Cx]
  [Gc] -> Habitacle4/3(Gc)
  Blé3/1(P_O2_b) -> 1-phi8/1, Scope46/1
  [P_CO2_c] -> Sum15/2, Scope53/1
  Sum12/1 -> Scope41/1, Habitacle4/1(P_O2_e)
  Habitacle4/1(P_O2_c) -> Scope38/1, To Workspace13/1, Blé3/1(P_O2_c), [P_O2_c], Scope44/1, Algue3/1(P_O2_c)
  phi8/1 -> Sum12/2
  Gain3/1 -> PID Controller3/1
  Sum11/1 -> Gain5/1
  PID Controller5/1 -> Saturation5/1
  PID Controller4/1 -> Saturation4/1
  Algue3/1(P_O2_a) -> phi8/1, Scope42/1
  phi9/1 -> Sum13/2
  Sum15/1 -> Gain4/1
  [phi0] -> Algue3/4(phi0)
  Algue3/2(P_CO2_a) -> Scope43/1, phi9/1
  Saturation4/1 -> To Workspace16/1, Scope52/1, [Gc]
  Step11/1 -> Goto17/1
  Habitacle4/2(P_CO2_c) -> To Workspace12/1, Scope39/1, [P_CO2_c], Scope45/1, Algue3/2(P_CO2_c), Blé3/2(P_CO2_c)
  [Cx] -> Sum14/2, Scope50/1
  Saturation3/1 -> Scope49/1, [Lr]
  Sum13/1 -> Scope40/1, Habitacle4/2(P_CO2_e)
  Blé3/2(P_CO2_b) -> 1-phi9/1, Scope47/1
  [Gc] -> Algue3/5(Gc)
  [P_O2_c] -> Sum11/2, Scope55/1
  Saturation5/1 -> To Workspace15/1, Scope54/1, [phi0]
  [Gc] -> Blé3/3(Gc)
  Gain5/1 -> PID Controller5/1
  Step14/1 -> Goto14/1
  Step16/1 -> Goto18/1
  [dotOmega_CO2] -> Habitacle4/4(dotOmega_CO2)
  [dotOmega_O2] -> Habitacle4/5(dotOmega_O2)
  Sum16/1 -> Scope56/1, [dotOmega_CO2]
  Step19/1 -> Sum16/2
  Step17/1 -> Sum16/1
  Step18/1 -> Sum17/1
  Step20/1 -> Sum17/2
  Sum17/1 -> Scope57/1, [dotOmega_O2]

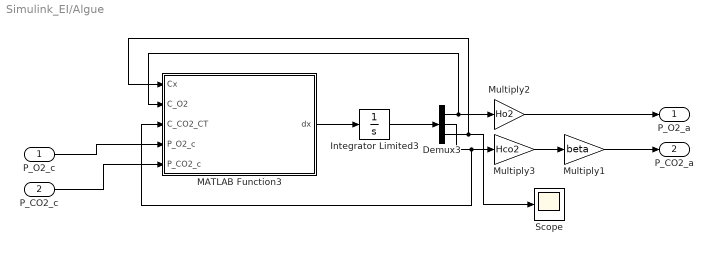
== system Simulink_EI/Algue ==
  P_O2_c : Inport
  P_CO2_c : Inport  Port=2
  Demux3 : Demux  Outputs=3
  Integrator Limited3 : Integrator  InitialCondition=[0.2118;8.50;1]  LimitOutput=on  LowerSaturationLimit=0
  MATLAB Function3 : MATLAB Function  TreatAsAtomicUnit=on
  Multiply1 : Gain  Gain=beta
  Multiply2 : Gain  Gain=Ho2
  Multiply3 : Gain  Gain=Hco2
  Scope : Scope
  P_O2_a : Outport
  P_CO2_a : Outport  Port=2
  wires:
  Demux3/2 -> MATLAB Function3/3(C_CO2_CT), Multiply3/1
  Demux3/1 -> MATLAB Function3/2(C_O2), Multiply2/1
  Integrator Limited3/1 -> Demux3/1
  Multiply3/1 -> Multiply1/1
  Demux3/3 -> Scope/1, MATLAB Function3/1(Cx)
  MATLAB Function3/1(dx) -> Integrator Limited3/1
  Multiply2/1 -> P_O2_a/1
  P_O2_c/1 -> MATLAB Function3/4(P_O2_c)
  P_CO2_c/1 -> MATLAB Function3/5(P_CO2_c)
  Multiply1/1 -> P_CO2_a/1

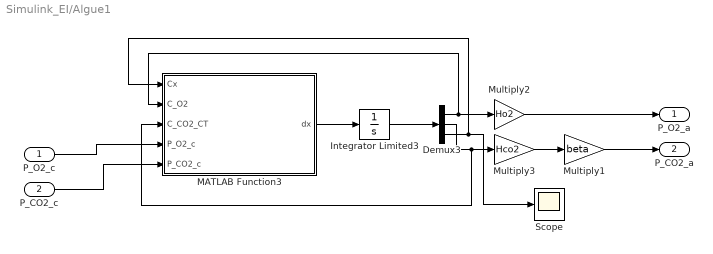
== system Simulink_EI/Algue1 ==
  P_O2_c : Inport
  P_CO2_c : Inport  Port=2
  Demux3 : Demux  Outputs=3
  Integrator Limited3 : Integrator  InitialCondition=[0.2118;8.50;1]  LimitOutput=on  LowerSaturationLimit=0
  MATLAB Function3 : MATLAB Function  TreatAsAtomicUnit=on
  Multiply1 : Gain  Gain=beta
  Multiply2 : Gain  Gain=Ho2
  Multiply3 : Gain  Gain=Hco2
  Scope : Scope
  P_O2_a : Outport
  P_CO2_a : Outport  Port=2
  wires:
  Demux3/2 -> MATLAB Function3/3(C_CO2_CT), Multiply3/1
  Demux3/1 -> MATLAB Function3/2(C_O2), Multiply2/1
  Integrator Limited3/1 -> Demux3/1
  Multiply3/1 -> Multiply1/1
  Demux3/3 -> Scope/1, MATLAB Function3/1(Cx)
  MATLAB Function3/1(dx) -> Integrator Limited3/1
  Multiply2/1 -> P_O2_a/1
  P_O2_c/1 -> MATLAB Function3/4(P_O2_c)
  P_CO2_c/1 -> MATLAB Function3/5(P_CO2_c)
  Multiply1/1 -> P_CO2_a/1

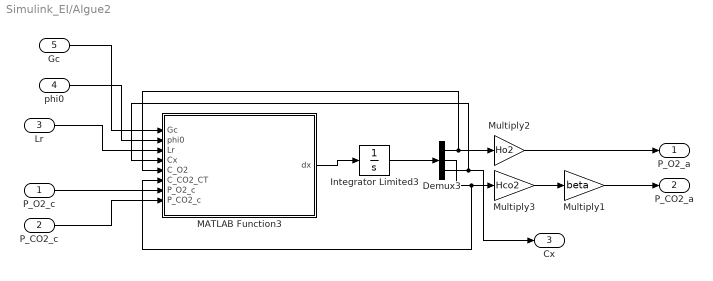
== system Simulink_EI/Algue2 ==
  P_O2_c : Inport
  P_CO2_c : Inport  Port=2
  Lr : Inport  Port=3
  phi0 : Inport  Port=4
  Gc : Inport  Port=5
  Demux3 : Demux  Outputs=3
  Integrator Limited3 : Integrator  InitialCondition=[0.2118;8.50;1]  LimitOutput=on  LowerSaturationLimit=0
  MATLAB Function3 : MATLAB Function  TreatAsAtomicUnit=on
  Multiply1 : Gain  Gain=beta
  Multiply2 : Gain  Gain=Ho2
  Multiply3 : Gain  Gain=Hco2
  P_O2_a : Outport
  P_CO2_a : Outport  Port=2
  Cx : Outport  Port=3
  wires:
  Demux3/2 -> MATLAB Function3/6(C_CO2_CT), Multiply3/1
  Demux3/1 -> MATLAB Function3/5(C_O2), Multiply2/1
  Integrator Limited3/1 -> Demux3/1
  Multiply3/1 -> Multiply1/1
  Demux3/3 -> Cx/1, MATLAB Function3/4(Cx)
  MATLAB Function3/1(dx) -> Integrator Limited3/1
  Multiply2/1 -> P_O2_a/1
  P_O2_c/1 -> MATLAB Function3/7(P_O2_c)
  P_CO2_c/1 -> MATLAB Function3/8(P_CO2_c)
  Multiply1/1 -> P_CO2_a/1
  Lr/1 -> MATLAB Function3/3(Lr)
  phi0/1 -> MATLAB Function3/2(phi0)
  Gc/1 -> MATLAB Function3/1(Gc)

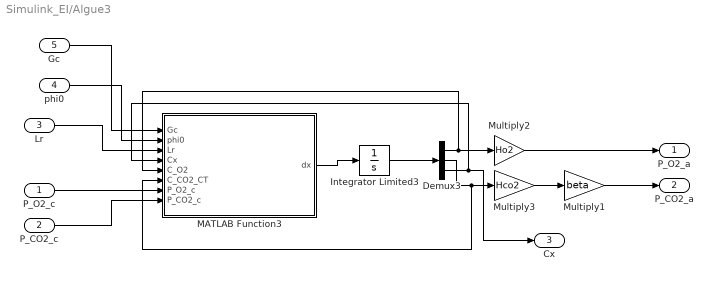
== system Simulink_EI/Algue3 ==
  P_O2_c : Inport
  P_CO2_c : Inport  Port=2
  Lr : Inport  Port=3
  phi0 : Inport  Port=4
  Gc : Inport  Port=5
  Demux3 : Demux  Outputs=3
  Integrator Limited3 : Integrator  InitialCondition=[0.2118;8.50;1]  LimitOutput=on  LowerSaturationLimit=0
  MATLAB Function3 : MATLAB Function  TreatAsAtomicUnit=on
  Multiply1 : Gain  Gain=beta
  Multiply2 : Gain  Gain=Ho2
  Multiply3 : Gain  Gain=Hco2
  P_O2_a : Outport
  P_CO2_a : Outport  Port=2
  Cx : Outport  Port=3
  wires:
  Demux3/2 -> MATLAB Function3/6(C_CO2_CT), Multiply3/1
  Demux3/1 -> MATLAB Function3/5(C_O2), Multiply2/1
  Integrator Limited3/1 -> Demux3/1
  Multiply3/1 -> Multiply1/1
  Demux3/3 -> Cx/1, MATLAB Function3/4(Cx)
  MATLAB Function3/1(dx) -> Integrator Limited3/1
  Multiply2/1 -> P_O2_a/1
  P_O2_c/1 -> MATLAB Function3/7(P_O2_c)
  P_CO2_c/1 -> MATLAB Function3/8(P_CO2_c)
  Multiply1/1 -> P_CO2_a/1
  Lr/1 -> MATLAB Function3/3(Lr)
  phi0/1 -> MATLAB Function3/2(phi0)
  Gc/1 -> MATLAB Function3/1(Gc)

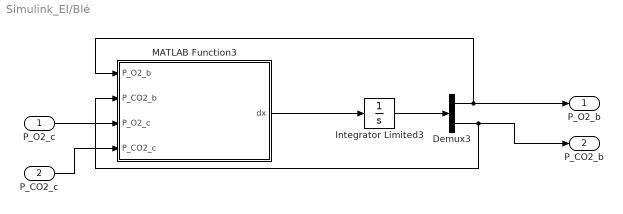
== system Simulink_EI/Blé ==
  P_O2_c : Inport
  P_CO2_c : Inport  Port=2
  Demux3 : Demux  Outputs=2
  Integrator Limited3 : Integrator  InitialCondition=[21247;20.35]  LimitOutput=on  LowerSaturationLimit=0
  MATLAB Function3 : MATLAB Function  TreatAsAtomicUnit=on
  P_O2_b : Outport
  P_CO2_b : Outport  Port=2
  wires:
  Demux3/1 -> MATLAB Function3/1(P_O2_b), P_O2_b/1
  Demux3/2 -> MATLAB Function3/2(P_CO2_b), P_CO2_b/1
  MATLAB Function3/1(dx) -> Integrator Limited3/1
  Integrator Limited3/1 -> Demux3/1
  P_O2_c/1 -> MATLAB Function3/3(P_O2_c)
  P_CO2_c/1 -> MATLAB Function3/4(P_CO2_c)

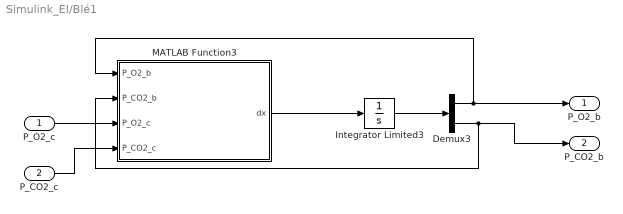
== system Simulink_EI/Blé1 ==
  P_O2_c : Inport
  P_CO2_c : Inport  Port=2
  Demux3 : Demux  Outputs=2
  Integrator Limited3 : Integrator  InitialCondition=[21247;20.35]  LimitOutput=on  LowerSaturationLimit=0
  MATLAB Function3 : MATLAB Function  TreatAsAtomicUnit=on
  P_O2_b : Outport
  P_CO2_b : Outport  Port=2
  wires:
  Demux3/1 -> MATLAB Function3/1(P_O2_b), P_O2_b/1
  Demux3/2 -> MATLAB Function3/2(P_CO2_b), P_CO2_b/1
  MATLAB Function3/1(dx) -> Integrator Limited3/1
  Integrator Limited3/1 -> Demux3/1
  P_O2_c/1 -> MATLAB Function3/3(P_O2_c)
  P_CO2_c/1 -> MATLAB Function3/4(P_CO2_c)

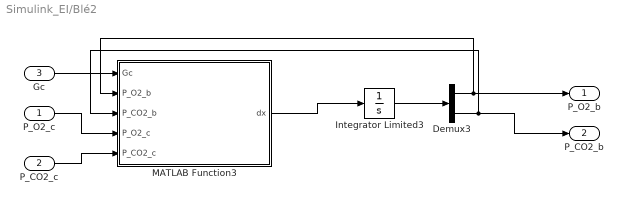
== system Simulink_EI/Blé2 ==
  P_O2_c : Inport
  P_CO2_c : Inport  Port=2
  Gc : Inport  Port=3
  Demux3 : Demux  Outputs=2
  Integrator Limited3 : Integrator  InitialCondition=[21247;20.35]  LimitOutput=on  LowerSaturationLimit=0
  MATLAB Function3 : MATLAB Function  TreatAsAtomicUnit=on
  P_O2_b : Outport
  P_CO2_b : Outport  Port=2
  wires:
  Demux3/1 -> MATLAB Function3/2(P_O2_b), P_O2_b/1
  Demux3/2 -> MATLAB Function3/3(P_CO2_b), P_CO2_b/1
  MATLAB Function3/1(dx) -> Integrator Limited3/1
  Integrator Limited3/1 -> Demux3/1
  P_O2_c/1 -> MATLAB Function3/4(P_O2_c)
  P_CO2_c/1 -> MATLAB Function3/5(P_CO2_c)
  Gc/1 -> MATLAB Function3/1(Gc)

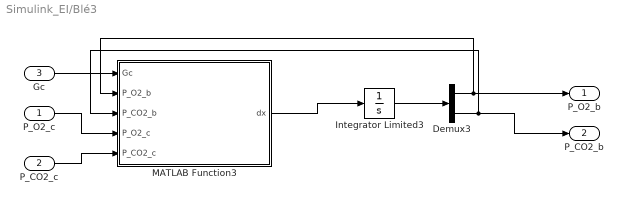
== system Simulink_EI/Blé3 ==
  P_O2_c : Inport
  P_CO2_c : Inport  Port=2
  Gc : Inport  Port=3
  Demux3 : Demux  Outputs=2
  Integrator Limited3 : Integrator  InitialCondition=[21247;20.35]  LimitOutput=on  LowerSaturationLimit=0
  MATLAB Function3 : MATLAB Function  TreatAsAtomicUnit=on
  P_O2_b : Outport
  P_CO2_b : Outport  Port=2
  wires:
  Demux3/1 -> MATLAB Function3/2(P_O2_b), P_O2_b/1
  Demux3/2 -> MATLAB Function3/3(P_CO2_b), P_CO2_b/1
  MATLAB Function3/1(dx) -> Integrator Limited3/1
  Integrator Limited3/1 -> Demux3/1
  P_O2_c/1 -> MATLAB Function3/4(P_O2_c)
  P_CO2_c/1 -> MATLAB Function3/5(P_CO2_c)
  Gc/1 -> MATLAB Function3/1(Gc)

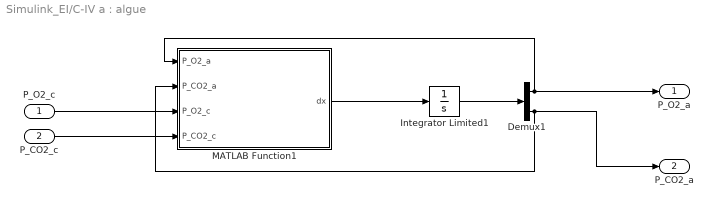
== system Simulink_EI/C-IV a : algue ==
  P_O2_c : Inport
  P_CO2_c : Inport  Port=2
  Demux1 : Demux  Outputs=2
  Integrator Limited1 : Integrator  LimitOutput=on  LowerSaturationLimit=0
  MATLAB Function1 : MATLAB Function  TreatAsAtomicUnit=on
  P_O2_a : Outport
  P_CO2_a : Outport  Port=2
  wires:
  Demux1/1 -> P_O2_a/1, MATLAB Function1/1(P_O2_a)
  MATLAB Function1/1(dx) -> Integrator Limited1/1
  Demux1/2 -> P_CO2_a/1, MATLAB Function1/2(P_CO2_a)
  Integrator Limited1/1 -> Demux1/1
  P_O2_c/1 -> MATLAB Function1/3(P_O2_c)
  P_CO2_c/1 -> MATLAB Function1/4(P_CO2_c)

== system Simulink_EI/C-IV b : blé ==
  P_O2_c : Inport
  P_CO2_c : Inport  Port=2
  Demux2 : Demux  Outputs=2
  Integrator Limited2 : Integrator  LimitOutput=on  LowerSaturationLimit=0
  MATLAB Function2 : MATLAB Function  TreatAsAtomicUnit=on
  P_O2_b : Outport
  P_CO2_b : Outport  Port=2
  wires:
  MATLAB Function2/1(dx) -> Integrator Limited2/1
  Integrator Limited2/1 -> Demux2/1
  P_O2_c/1 -> MATLAB Function2/3(P_O2_c)
  P_CO2_c/1 -> MATLAB Function2/4(P_CO2_c)
  Demux2/2 -> MATLAB Function2/2(P_CO2_b), P_CO2_b/1
  Demux2/1 -> MATLAB Function2/1(P_O2_b), P_O2_b/1

== system Simulink_EI/Habitacle ==
  P_O2_e : Inport
  P_CO2_e : Inport  Port=2
  Demux : Demux  Outputs=2
  Integrator Limited : Integrator  LimitOutput=on  LowerSaturationLimit=0
  MATLAB Function : MATLAB Function  TreatAsAtomicUnit=on
  P_O2_c : Outport
  P_CO2_c : Outport  Port=2
  wires:
  Demux/2 -> P_CO2_c/1, MATLAB Function/2(P_CO2_c)
  Integrator Limited/1 -> Demux/1
  Demux/1 -> P_O2_c/1, MATLAB Function/1(P_O2_c)
  MATLAB Function/1(dx) -> Integrator Limited/1
  P_CO2_e/1 -> MATLAB Function/4(P_CO2_e)
  P_O2_e/1 -> MATLAB Function/3(P_O2_e)

== system Simulink_EI/Habitacle1 ==
  P_O2_e : Inport
  P_CO2_e : Inport  Port=2
  Demux3 : Demux  Outputs=2
  Integrator Limited3 : Integrator  InitialCondition=[20000;40]  LimitOutput=on  LowerSaturationLimit=0
  MATLAB Function3 : MATLAB Function  TreatAsAtomicUnit=on
  P_O2_c : Outport
  P_CO2_c : Outport  Port=2
  wires:
  MATLAB Function3/1(dx) -> Integrator Limited3/1
  Integrator Limited3/1 -> Demux3/1
  Demux3/1 -> MATLAB Function3/1(P_O2_c), P_O2_c/1
  P_O2_e/1 -> MATLAB Function3/3(P_O2_e)
  P_CO2_e/1 -> MATLAB Function3/4(P_CO2_e)
  Demux3/2 -> MATLAB Function3/2(P_CO2_c), P_CO2_c/1

== system Simulink_EI/Habitacle2 ==
  P_O2_e : Inport
  P_CO2_e : Inport  Port=2
  Demux3 : Demux  Outputs=2
  Integrator Limited3 : Integrator  InitialCondition=[20000;40]  LimitOutput=on  LowerSaturationLimit=0
  MATLAB Function3 : MATLAB Function  TreatAsAtomicUnit=on
  P_O2_c : Outport
  P_CO2_c : Outport  Port=2
  wires:
  MATLAB Function3/1(dx) -> Integrator Limited3/1
  Integrator Limited3/1 -> Demux3/1
  Demux3/1 -> MATLAB Function3/1(P_O2_c), P_O2_c/1
  P_O2_e/1 -> MATLAB Function3/3(P_O2_e)
  P_CO2_e/1 -> MATLAB Function3/4(P_CO2_e)
  Demux3/2 -> MATLAB Function3/2(P_CO2_c), P_CO2_c/1

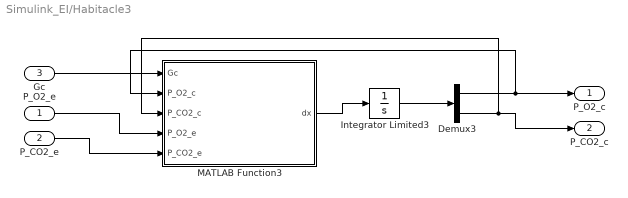
== system Simulink_EI/Habitacle3 ==
  P_O2_e : Inport
  P_CO2_e : Inport  Port=2
  Gc : Inport  Port=3
  Demux3 : Demux  Outputs=2
  Integrator Limited3 : Integrator  InitialCondition=[20000;40]  LimitOutput=on  LowerSaturationLimit=0
  MATLAB Function3 : MATLAB Function  TreatAsAtomicUnit=on
  P_O2_c : Outport
  P_CO2_c : Outport  Port=2
  wires:
  MATLAB Function3/1(dx) -> Integrator Limited3/1
  Integrator Limited3/1 -> Demux3/1
  Demux3/1 -> MATLAB Function3/2(P_O2_c), P_O2_c/1
  P_O2_e/1 -> MATLAB Function3/4(P_O2_e)
  P_CO2_e/1 -> MATLAB Function3/5(P_CO2_e)
  Demux3/2 -> MATLAB Function3/3(P_CO2_c), P_CO2_c/1
  Gc/1 -> MATLAB Function3/1(Gc)

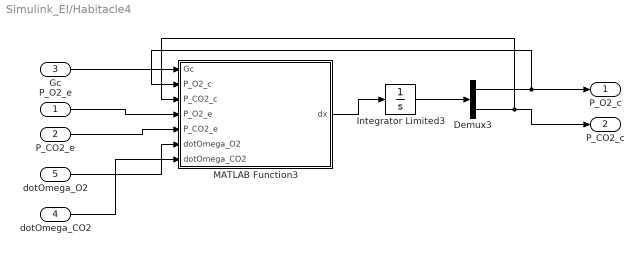
== system Simulink_EI/Habitacle4 ==
  P_O2_e : Inport
  P_CO2_e : Inport  Port=2
  Gc : Inport  Port=3
  dotOmega_CO2 : Inport  Port=4
  dotOmega_O2 : Inport  Port=5
  Demux3 : Demux  Outputs=2
  Integrator Limited3 : Integrator  InitialCondition=[20000;40]  LimitOutput=on  LowerSaturationLimit=0
  MATLAB Function3 : MATLAB Function  TreatAsAtomicUnit=on
  P_O2_c : Outport
  P_CO2_c : Outport  Port=2
  wires:
  MATLAB Function3/1(dx) -> Integrator Limited3/1
  Integrator Limited3/1 -> Demux3/1
  Demux3/1 -> MATLAB Function3/2(P_O2_c), P_O2_c/1
  P_O2_e/1 -> MATLAB Function3/4(P_O2_e)
  P_CO2_e/1 -> MATLAB Function3/5(P_CO2_e)
  Demux3/2 -> MATLAB Function3/3(P_CO2_c), P_CO2_c/1
  Gc/1 -> MATLAB Function3/1(Gc)
  dotOmega_O2/1 -> MATLAB Function3/6(dotOmega_O2)
  dotOmega_CO2/1 -> MATLAB Function3/7(dotOmega_CO2)

== matlab function Simulink_EI/Blé/MATLAB Function3 ==
  data: P_O2_b input; P_CO2_b input; P_O2_c input; P_CO2_c input; dx output
function dx = ble(P_O2_b,P_CO2_b,P_O2_c,P_CO2_c)

Gc = 13680;
R  = 8.314;    % [J/(mol·K)]
Tb  = 296;      % [K] 
S = 44.98;
phi = 0.2029;
Vb = S;
T_ref = 298;

H = 20;            % Durée d'ensoleillement en heures (à définir)
C = 0.68;          % Coefficient d'efficacité (à définir)
A_max = 0.93;        % Surface maximale (à définir)
F = 1.4*10^(-3)*24*3600;            % Facteur de flux (à définir)
t_q = 33;          % Durée de photosynthèse active (à définir)
t_a = 12;      % Temps de démarrage de la photosynthèse (à définir)
t_m = 62;          % Durée totale de mesure (à définir)

q_max = 0.05 + 1.437e-4 * (P_CO2_b - 33);
q_min = 0.01 + 2.87e-5 * (P_CO2_b - 33);
P_g = 0.5 * A_max * F * (q_max * (1 + (t_q - t_a) / t_m) + q_min * (1 - t_q / t_m));

dx = zeros(2,1);

P_24_j = (H*C*P_g/24) + (1-C)*4*P_g/24;

k1 = (1-phi)*Gc*Tb / (Vb*T_ref);
k2 = P_24_j*R*Tb*S / Vb;

dx(1) = k1 * (P_O2_c - P_O2_b) + k2 ;   
dx(2) = k1 * (P_CO2_c - P_CO2_b) - k2;

== matlab function Simulink_EI/Algue1/MATLAB Function3 ==
  data: Cx input; C_O2 input; C_CO2_CT input; P_O2_c input; P_CO2_c input; dx output
function dx = algue(Cx,C_O2,C_CO2_CT,P_O2_c,P_CO2_c)

Gc = 13680;
R  = 8.314;    % [J/(mol·K)]
Vl = 0.384;
phi = 0.2029;
Qp = 1.4285;
H_O2 = 94565;
H_CO2 = 4003;
Mx = 0.0222;
beta = 1/1820.89;
phi0 = 350;
L = 0.018;
m = 310;
mu_M = 0.143*24;
KJ = 40;
T_ref = 298;

Lr = 0.52992;

L2 = log(phi0) / (m * Cx);
Lmin = min(L2, L);
rx = (mu_M / (m*L)) * log( (phi0 + KJ) / (phi0 * exp(-m * Cx * Lmin) + KJ) );

dx = zeros(3,1);

k1 = phi*Gc / (Vl*R*T_ref);
k2 = rx/Mx;

dx(1) = k1 * (P_O2_c - H_O2*C_O2) + k2 * Qp;   
dx(2) = k1 * (P_CO2_c - H_CO2*C_CO2_CT*beta) - k2;  
dx(3) = rx - Lr*Cx/Vl;

== matlab function Simulink_EI/Blé1/MATLAB Function3 ==
  data: P_O2_b input; P_CO2_b input; P_O2_c input; P_CO2_c input; dx output
function dx = ble(P_O2_b,P_CO2_b,P_O2_c,P_CO2_c)

Gc = 13680;
R  = 8.314;    % [J/(mol·K)]
Tb  = 296;      % [K] 
S = 44.98;
phi = 0.2029;
Vb = S;
T_ref = 298;

H = 20;            % Durée d'ensoleillement en heures (à définir)
C = 0.68;          % Coefficient d'efficacité (à définir)
A_max = 0.93;        % Surface maximale (à définir)
F = 1.4*10^(-3)*24*3600;            % Facteur de flux (à définir)
t_q = 33;          % Durée de photosynthèse active (à définir)
t_a = 12;      % Temps de démarrage de la photosynthèse (à définir)
t_m = 62;          % Durée totale de mesure (à définir)

q_max = 0.05 + 1.437e-4 * (P_CO2_b - 33);
q_min = 0.01 + 2.87e-5 * (P_CO2_b - 33);
P_g = 0.5 * A_max * F * (q_max * (1 + (t_q - t_a) / t_m) + q_min * (1 - t_q / t_m));

dx = zeros(2,1);

P_24_j = (H*C*P_g/24) + (1-C)*4*P_g/24;

k1 = (1-phi)*Gc*Tb / (Vb*T_ref);
k2 = P_24_j*R*Tb*S / Vb;

dx(1) = k1 * (P_O2_c - P_O2_b) + k2 ;   
dx(2) = k1 * (P_CO2_c - P_CO2_b) - k2;

== matlab function Simulink_EI/Habitacle2/MATLAB Function3 ==
  data: P_O2_c input; P_CO2_c input; dx output; P_O2_e input; P_CO2_e input
function dx = Habitacle(P_O2_c,P_CO2_c,P_O2_e,P_CO2_e)

Gc = 13680;     
Vc = 125;    % [m³]
R  = 8.314;    % [J/(mol·K)]
Tc  = 296;      % [K]
Np = 5;      
dotOmega_O2 = -1.065*24;
dotOmega_CO2 =  0.982*24;
T_ref = 298;

dx = zeros(2,1);

k1 = Gc*Tc / (Vc*T_ref);
k2 = R * Tc * Np / Vc;

dx(1) = k1 * (P_O2_e - P_O2_c) + k2 * dotOmega_O2;   % dP_O2^c / dt
dx(2) = k1 * (P_CO2_e - P_CO2_c) + k2 * dotOmega_CO2;   % dP_CO2^c / dt

== matlab function Simulink_EI/Algue2/MATLAB Function3 ==
  data: Gc input; phi0 input; Lr input; Cx input; C_O2 input; C_CO2_CT input; P_O2_c input; P_CO2_c input; dx output
function dx = algue(Gc,phi0,Lr,Cx,C_O2,C_CO2_CT,P_O2_c,P_CO2_c)

%Gc = 13680;
R  = 8.314;    % [J/(mol·K)]
Vl = 0.384;
phi = 0.2029;
Qp = 1.4285;
H_O2 = 94565;
H_CO2 = 4003;
Mx = 0.0222;
beta = 1/1820.89;
L = 0.018;
m = 310;
mu_M = 0.143*24;
KJ = 40;
T_ref = 298;

L2 = log(phi0) / (m * Cx);
Lmin = min(L2, L);
rx = (mu_M / (m*L)) * log( (phi0 + KJ) / (phi0 * exp(-m * Cx * Lmin) + KJ) );

dx = zeros(3,1);

k1 = phi*Gc / (Vl*R*T_ref);
k2 = rx/Mx;

dx(1) = k1 * (P_O2_c - H_O2*C_O2) + k2 * Qp;   
dx(2) = k1 * (P_CO2_c - H_CO2*C_CO2_CT*beta) - k2;  
dx(3) = rx - Lr*Cx/Vl;

== matlab function Simulink_EI/Blé2/MATLAB Function3 ==
  data: Gc input; P_O2_b input; P_CO2_b input; P_O2_c input; P_CO2_c input; dx output
function dx = ble(Gc,P_O2_b,P_CO2_b,P_O2_c,P_CO2_c)

%Gc = 13680;
R  = 8.314;    % [J/(mol·K)]
Tb  = 296;      % [K] 
S = 44.98;
phi = 0.2029;
Vb = S;
T_ref = 298;

H = 20;            % Durée d'ensoleillement en heures (à définir)
C = 0.68;          % Coefficient d'efficacité (à définir)
A_max = 0.93;        % Surface maximale (à définir)
F = 1.4*10^(-3)*24*3600;            % Facteur de flux (à définir)
t_q = 33;          % Durée de photosynthèse active (à définir)
t_a = 12;      % Temps de démarrage de la photosynthèse (à définir)
t_m = 62;          % Durée totale de mesure (à définir)

q_max = 0.05 + 1.437e-4 * (P_CO2_b - 33);
q_min = 0.01 + 2.87e-5 * (P_CO2_b - 33);
P_g = 0.5 * A_max * F * (q_max * (1 + (t_q - t_a) / t_m) + q_min * (1 - t_q / t_m));

dx = zeros(2,1);

P_24_j = (H*C*P_g/24) + (1-C)*4*P_g/24;

k1 = (1-phi)*Gc*Tb / (Vb*T_ref);
k2 = P_24_j*R*Tb*S / Vb;

dx(1) = k1 * (P_O2_c - P_O2_b) + k2 ;   
dx(2) = k1 * (P_CO2_c - P_CO2_b) - k2;

== matlab function Simulink_EI/Habitacle3/MATLAB Function3 ==
  data: Gc input; P_O2_c input; P_CO2_c input; dx output; P_O2_e input; P_CO2_e input
function dx = Habitacle(Gc,P_O2_c,P_CO2_c,P_O2_e,P_CO2_e)

%Gc = 13680;     
Vc = 125;    % [m³]
R  = 8.314;    % [J/(mol·K)]
Tc  = 296;      % [K]
Np = 5;      
dotOmega_O2 = -1.065*24;
dotOmega_CO2 =  0.982*24;
T_ref = 298;

dx = zeros(2,1);

k1 = Gc*Tc / (Vc*T_ref);
k2 = R * Tc * Np / Vc;

dx(1) = k1 * (P_O2_e - P_O2_c) + k2 * dotOmega_O2;   % dP_O2^c / dt
dx(2) = k1 * (P_CO2_e - P_CO2_c) + k2 * dotOmega_CO2;   % dP_CO2^c / dt

== matlab function Simulink_EI/Algue3/MATLAB Function3 ==
  data: Gc input; phi0 input; Lr input; Cx input; C_O2 input; C_CO2_CT input; P_O2_c input; P_CO2_c input; dx output
function dx = algue(Gc,phi0,Lr,Cx,C_O2,C_CO2_CT,P_O2_c,P_CO2_c)

%Gc = 13680;
R  = 8.314;    % [J/(mol·K)]
Vl = 0.384;
phi = 0.2029;
Qp = 1.4285;
H_O2 = 94565;
H_CO2 = 4003;
Mx = 0.0222;
beta = 1/1820.89;
L = 0.018;
m = 310;
mu_M = 0.143*24;
KJ = 40;
T_ref = 298;

L2 = log(phi0) / (m * Cx);
Lmin = min(L2, L);
rx = (mu_M / (m*L)) * log( (phi0 + KJ) / (phi0 * exp(-m * Cx * Lmin) + KJ) );

dx = zeros(3,1);

k1 = phi*Gc / (Vl*R*T_ref);
k2 = rx/Mx;

dx(1) = k1 * (P_O2_c - H_O2*C_O2) + k2 * Qp;   
dx(2) = k1 * (P_CO2_c - H_CO2*C_CO2_CT*beta) - k2;  
dx(3) = rx - Lr*Cx/Vl;
